simulink model "SimulacionesI"  (Simulink 8.9)
settings: Solver=VariableStepAuto  StartTime=0.0  StopTime=1000  RelTol=1e-3
values from neighbouring files (symbols this model uses):
  B = 2*((psi*wn)^2)*I3    (= 6.76461887388e-07)    [Simulaciones.m]
  FrecRuido = wcHz*100    (= 15.9154943092)    [Simulaciones.m]
  Fs = 3*FrecRuidoBloque    (= 95.4929658551)    [Simulaciones.m]
  Is = 1e3    (= 1000)    [Simulaciones.m]
  K = Is*wn^2    (= 0.1)    [Simulaciones.m]
  Kd = 2*psi*wn*Is    (= 14)    [Simulaciones.m]
  wc = wn*100    (= 1)    [Simulaciones.m]
libraries: simulink x4
settings Model: SuppressorTable=22 serialization::archive 11 0 6 0 0 0 11 0  Creator=root  LastModifiedBy=root
settings DataIOCC: LimitDataPoints=off  SaveFormat=Dataset  SignalLoggingSaveFormat=Dataset
settings OptimizationCC: LifeSpan=auto
settings DebuggingCC: UnderspecifiedInitializationDetection=Simplified  MergeDetectMultiDrivingBlocksExec=error  FcnCallInpInsideContextMsg=error  StateNameClashWarn=none  SFUnexpectedBacktrackingDiag=error  SFNoUnconditionalDefaultTransitionDiag=error  SFExecutionAtInitializationDiag=warning
settings HardwareCC: ProdBitPerPointer=64  ProdBitPerSizeT=64  ProdBitPerPtrDiffT=64  ProdLargestAtomicFloat=Float  ProdIntDivRoundTo=Zero  ProdEndianess=LittleEndian  ProdWordSize=64  ProdHWDeviceType=Intel->x86-64 (Windows64)
settings ModelReferenceCC: PropagateSignalLabelsOutOfModel=on
settings GRTTargetCC: TargetLangStandard=C99 (ISO)  GeneratePreprocessorConditionals=Use local settings  CombineOutputUpdateFcns=on  GRTInterface=off
settings ConfigComp: CovMetricSettings=dwe  CovHtmlReporting=off  CovSaveCumulativeToWorkspaceVar=off  CovSaveSingleToWorkspaceVar=off  CovExternalEMLEnable=on

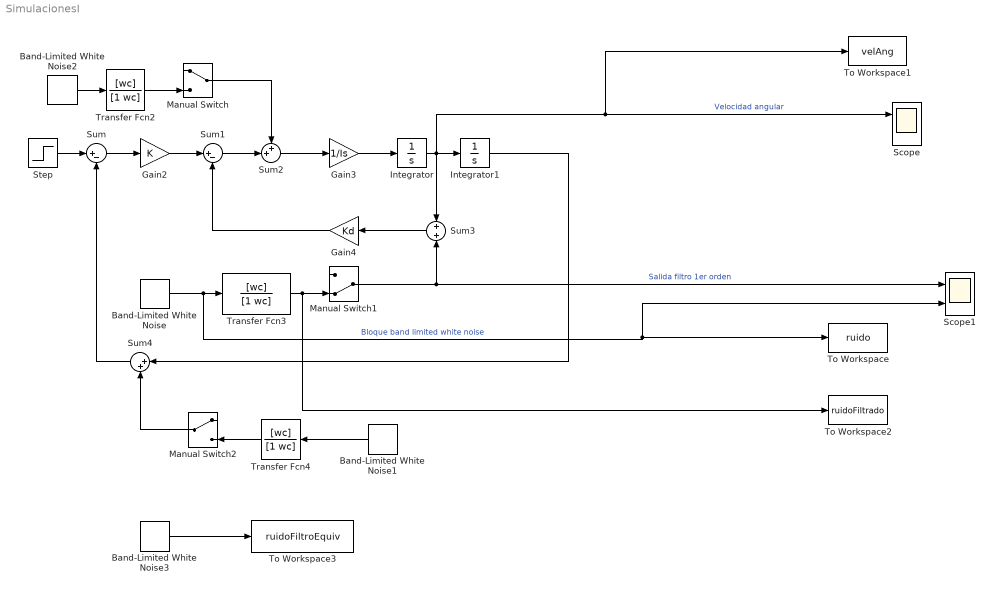
== system SimulacionesI ==
  Band-Limited White Noise : simulink/Sources/Band-Limited White Noise  Cov=A  Ts=1/FrecRuido  seed=[23341]
  Band-Limited White Noise1 : simulink/Sources/Band-Limited White Noise  Cov=A  Ts=1/FrecRuido  seed=[23341]
  Band-Limited White Noise2 : simulink/Sources/Band-Limited White Noise  Cov=A  Ts=1/FrecRuido  seed=[23341]
  Band-Limited White Noise3 : simulink/Sources/Band-Limited White Noise  Cov=A  Ts=1/B  seed=[23341]
  Gain2 : Gain  Gain=K
  Gain3 : Gain  Gain=1/Is
  Gain4 : Gain  Gain=Kd
  Integrator : Integrator
  Integrator1 : Integrator
  Manual Switch : ManualSwitch
  Manual Switch1 : ManualSwitch  CurrentSetting=0
  Manual Switch2 : ManualSwitch
  Scope : Scope  NumInputPorts=2
  Scope1 : Scope  NumInputPorts=2
  Step : Step  After=0  SampleTime=0
  Sum : Sum  Inputs=|+-
  Sum1 : Sum  Inputs=|+-
  Sum2 : Sum  Inputs=++|
  Sum3 : Sum  Inputs=+|+
  Sum4 : Sum  Inputs=|++
  To Workspace : ToWorkspace  VariableName=ruido  SaveFormat=Timeseries  SampleTime=1/Fs
  To Workspace1 : ToWorkspace  VariableName=velAng  SaveFormat=Timeseries  SampleTime=1/Fs
  To Workspace2 : ToWorkspace  VariableName=ruidoFiltrado  SaveFormat=Timeseries  SampleTime=1/Fs
  To Workspace3 : ToWorkspace  VariableName=ruidoFiltroEquiv  SaveFormat=Timeseries  SampleTime=1/Fs
  Transfer Fcn2 : TransferFcn  Numerator=[wc]  Denominator=[1 wc]
  Transfer Fcn3 : TransferFcn  Numerator=[wc]  Denominator=[1 wc]
  Transfer Fcn4 : TransferFcn  Numerator=[wc]  Denominator=[1 wc]
  wires:
  Gain3/1 -> Integrator/1
  Sum3/1 -> Gain4/1
  Integrator1/1 -> Sum4/1
  Sum4/1 -> Sum/2
  Sum/1 -> Gain2/1
  Gain2/1 -> Sum1/1
  Sum1/1 -> Sum2/2
  Sum2/1 -> Gain3/1
  Gain4/1 -> Sum1/2
  Transfer Fcn2/1 -> Manual Switch/2
  Manual Switch/1 -> Sum2/1
  Transfer Fcn3/1 -> To Workspace2/1, Manual Switch1/2
  Transfer Fcn4/1 -> Manual Switch2/2
  Manual Switch2/1 -> Sum4/2
  Step/1 -> Sum/1
  Band-Limited White Noise1/1 -> Transfer Fcn4/1
  Band-Limited White Noise2/1 -> Transfer Fcn2/1
  Integrator/1 -> Scope/1, To Workspace1/1, Sum3/1, Integrator1/1  "Velocidad angular"
  Manual Switch1/1 -> Scope1/1, Sum3/2  "Salida filtro 1er orden"
  Band-Limited White Noise/1 -> Transfer Fcn3/1, Scope1/2, To Workspace/1  "Bloque band limited white noise"
  Band-Limited White Noise3/1 -> To Workspace3/1
